simulink model "Sim"  (Simulink 9.3)
settings: Solver=ode45  StartTime=0.0  StopTime=20  RelTol=1e-5  EnableMultiTasking=on
settings Model: Creator=hp  LastModifiedBy=Edison  ExtModeTrigMode=oneshot  ExtModeArmWhenConnect=off
settings DataIOCC: SignalLoggingName=sigsOut
settings OptimizationCC: BooleanDataType=off  ExpressionDepthLimit=2147483647  InitFltsAndDblsToZero=on
settings DebuggingCC: SaveWithParameterizedLinksMsg=none  SignalResolutionControl=TryResolveAllWithWarning  MultiTaskDSMMsg=warning  MultiTaskCondExecSysMsg=none  StateNameClashWarn=warning
settings HardwareCC: TargetUnknown=on
settings SFSimCC: SimUseLocalCustomCode=on
settings RTWCC: RTWUseLocalCustomCode=on
settings GRTTargetCC: TargetFcnLib=ansi_tfl_tmw.mat
settings ConfigComp: CovExternalEMLEnable=on

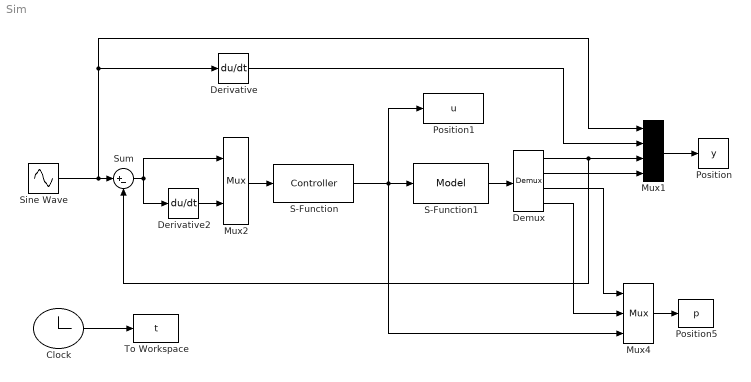
== system Sim ==
  Clock : Clock
  Demux : Demux
  Derivative : Derivative
  Derivative2 : Derivative
  Mux1 : Mux
  Mux2 : Mux  Inputs=2
  Mux4 : Mux  Inputs=3
  Position : ToWorkspace  VariableName=y  SampleTime=-1
  Position1 : ToWorkspace  VariableName=u  SampleTime=-1
  Position5 : ToWorkspace  VariableName=p  SampleTime=-1
  S-Function : S-Function  FunctionName=Controller  SFunctionDeploymentMode=off  EnableBusSupport=off
  S-Function1 : S-Function  FunctionName=Model  SFunctionDeploymentMode=off  EnableBusSupport=off
  Sine Wave : Sin  SampleTime=0
  Sum : Sum  Inputs=|+-  SaturateOnIntegerOverflow=on
  To Workspace : ToWorkspace  VariableName=t  SampleTime=-1
  wires:
  Mux1/1 -> Position/1
  Demux/1 -> Sum/2, Mux1/3
  S-Function1/1 -> Demux/1
  Clock/1 -> To Workspace/1
  Mux4/1 -> Position5/1
  Sine Wave/1 -> Sum/1, Mux1/1, Derivative/1
  Mux2/1 -> S-Function/1
  Sum/1 -> Mux2/1, Derivative2/1
  Derivative2/1 -> Mux2/2
  Demux/3 -> Mux4/1
  S-Function/1 -> S-Function1/1, Position1/1, Mux4/3
  Demux/4 -> Mux4/2
  Demux/2 -> Mux1/4
  Derivative/1 -> Mux1/2
